simulink library "aileronCtrl_ul"  (R2020a)
settings: Solver=VariableStepAuto  StartTime=0.0  StopTime=10.0  RelTol=1e-3
settings Model: Creator=Ayaz  LastModifiedBy=Ayaz

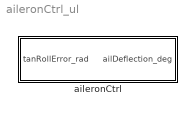
== system aileronCtrl_ul ==
  aileronCtrl : Subsystem  mask{ail_kp=0, ail_kd=0, ail_tau=0}
      mask prompts: ail_kp "Aileron kp [deg/deg]"; ail_kd "Aileron kd [deg/deg/s]"; ail_tau "Time constant [s]"

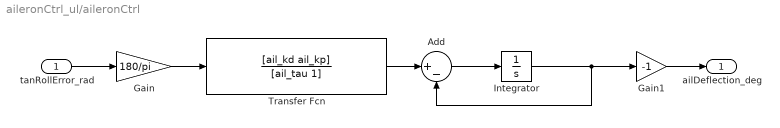
== system aileronCtrl_ul/aileronCtrl ==
  tanRollError_rad : Inport
  Add : Sum  Inputs=|+-
  Gain : Gain  Gain=180/pi
  Gain1 : Gain  Gain=-1
  Integrator : Integrator
  Transfer Fcn : TransferFcn  Numerator=[ail_kd ail_kp]  Denominator=[ail_tau 1]
  ailDeflection_deg : Outport
  wires:
  tanRollError_rad/1 -> Gain/1
  Gain/1 -> Transfer Fcn/1
  Transfer Fcn/1 -> Add/1
  Add/1 -> Integrator/1
  Integrator/1 -> Add/2, Gain1/1
  Gain1/1 -> ailDeflection_deg/1
